simulink model "model_linear"  (R2021b)
settings: Solver=VariableStepAuto  StartTime=0.0  StopTime=10  RelTol=1e-3
undefined symbols (not defined in the file): D, J, ke, Kp, L, P, Q, R, Tp, U
libraries: slpidlib x1
settings Model: Creator=mateusz  LastModifiedBy=mateusz

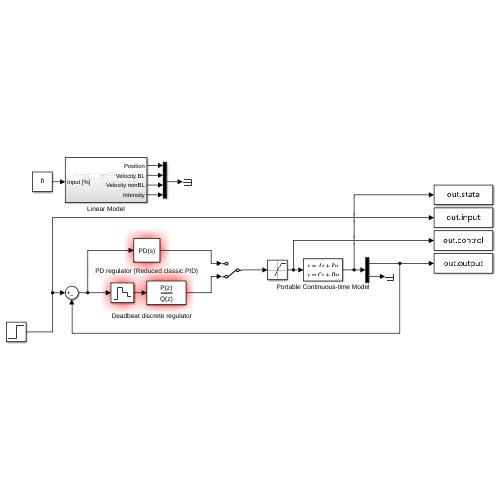
[thumbnail: Simulink's stored preview of the top-level diagram]
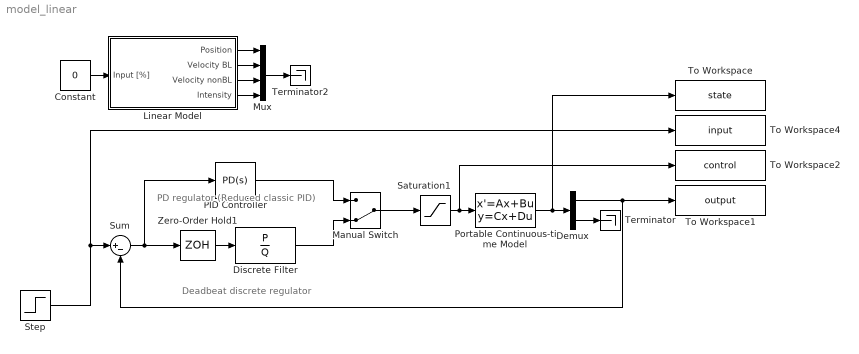
== system model_linear ==
  note: Deadbeat discrete regulator
  note: PD regulator (Reduced classic PID)
  Constant : Constant  Value=0
  Demux : Demux  Outputs=2
  Discrete Filter : DiscreteFilter  Numerator=P  Denominator=Q
  Linear Model : Subsystem
  Manual Switch : ManualSwitch  CurrentSetting=0
  Mux : Mux
  PID Controller : slpidlib/PID Controller  Controller=PD  Form=Parallel  TimeDomain=Continuous-time  UseExternalTs=off  SampleTime=-1  IntegratorMethod=Forward Euler  FilterMethod=Forward Euler  ControllerParametersSource=internal  P=Kp  I=0.000002  D=.667*Kp  UseFilter=on  N=100  TunerSelectOption=Transfer Function Based (PID Tuner App)  InitialConditionSource=internal  InitialConditionForIntegrator=0  InitialConditionForFilter=0  DifferentiatorICPrevScaledInput=0  ExternalReset=none  TrackingMode=off  Kt=1  LimitOutput=off  SatLimitsSource=internal  UpperSaturationLimit=inf  LowerSaturationLimit=-inf  LinearizeAsGain=on  AntiWindupMode=none  Kb=1  POutMin=[]  POutMax=[]  IOutMin=[]  IOutMax=[]  DOutMin=[]  DOutMax=[]  NOutMin=[]  NOutMax=[]  SumOutMin=[]  SumOutMax=[]  SaturationOutMin=[]  SaturationOutMax=[]  PParamMin=[]  PParamMax=[]  IParamMin=[]  IParamMax=[]  DParamMin=[]  DParamMax=[]  NParamMin=[]  NParamMax=[]  KbParamMin=[]  KbParamMax=[]  KtParamMin=[]  KtParamMax=[]  KbOutMin=[]  KbOutMax=[]  KtOutMin=[]  KtOutMax=[]  IntegratorOutMin=[]  IntegratorOutMax=[]  FilterOutMin=[]  FilterOutMax=[]  SumI1OutMin=[]  SumI1OutMax=[]  SumI2OutMin=[]  SumI2OutMax=[]  SumI3OutMin=[]  SumI3OutMax=[]  SumI4OutMin=[]  SumI4OutMax=[]  SumDOutMin=[]  SumDOutMax=[]  DifferentiatorOutMin=[]  DifferentiatorOutMax=[]  FilterDiffOutCoefMin=[]  FilterDiffOutCoefMax=[]  ReciprocalOutMin=[]  ReciprocalOutMax=[]  SumDenOutMin=[]  SumDenOutMax=[]  SumNumOutMin=[]  SumNumOutMax=[]  DivideOutMin=[]  DivideOutMax=[]  UdiffTsProdOutMin=[]  UdiffTsProdOutMax=[]  NTsProdOutMin=[]  NTsProdOutMax=[]  UintegralTsProdOutMin=[]  UintegralTsProdOutMax=[]  UngainTsProdOutMin=[]  UngainTsProdOutMax=[]  IntegratorContinuousStateAttributes=''  IntegratorStateMustResolveToSignalObject=off  IntegratorRTWStateStorageClass=Auto  FilterContinuousStateAttributes=''  FilterStateMustResolveToSignalObject=off  FilterRTWStateStorageClass=Auto  ParallelPVariant=InternalParameters  IdealPVariant=Disabled  IVariant=Disabled  DVariant=InternalParameters  IntegratorVariant=Disabled  SatVariant=Disabled  AWVariant=Disabled  PCopyVariant=Disabled  TRVariant=Disabled  FdbkBlocksVariant=Forward  IdealPFdbkVariant=Disabled  SatFdbkVariant=Disabled  DerivativeFilterVariant=ContFilter  NVariant=InternalParameters  NCopyVariant=Disabled  FilterICVariant=InternalICsFilter  IntegratorICVariant=Disabled  ExternalResetVariant=Disabled  TRSumVariant=Passthrough  SumFdbkVariant=Disabled  SumVariant=Sum_PD  TsampFilterVariant=InternalTs  TsampNgainVariant=Passthrough  TsampIntegralVariant=Disabled_SignalSpec  ExternalSaturationOutDataTypeStr=Inherit: Same as second input
  Portable Continuous-time Model : StateSpace  A=|  B=[0;0;0;2.59e4];  C=eye(4,4)  D=zeros(4,1)  InitialCondition=0
      | [0  1  0    0;
      |      0 -5  4.5  0;
      |      0  0 -0.7108*2  2*23.6012;
      |      0  0 -5.3898 -4040];
  Saturation1 : Saturate
  Step : Step  Time=0.5  After=6.28*25  SampleTime=0
  Sum : Sum  Inputs=|+-
  Terminator : Terminator
  Terminator2 : Terminator
  To Workspace : ToWorkspace  VariableName=state  SampleTime=-1
  To Workspace1 : ToWorkspace  VariableName=output  SampleTime=-1
  To Workspace2 : ToWorkspace  VariableName=control  SaveFormat=Structure With Time  SampleTime=0.001
  To Workspace4 : ToWorkspace  VariableName=input  SaveFormat=Structure With Time  SampleTime=-1
  Zero-Order Hold1 : ZeroOrderHold  SampleTime=Tp
  wires:
  Constant/1 -> Linear Model/1(Input [%])
  Linear Model/1(Position) -> Mux/1
  Linear Model/2(Velocity BL) -> Mux/2
  Linear Model/3(Velocity nonBL) -> Mux/3
  Linear Model/4(Intensity) -> Mux/4
  Portable Continuous-time Model/1 -> To Workspace/1, Demux/1
  Demux/1 -> To Workspace1/1, Sum/2
  Demux/2 -> Terminator/1
  Mux/1 -> Terminator2/1
  PID Controller/1 -> Manual Switch/1
  Zero-Order Hold1/1 -> Discrete Filter/1
  Manual Switch/1 -> Saturation1/1
  Discrete Filter/1 -> Manual Switch/2
  Saturation1/1 -> To Workspace2/1, Portable Continuous-time Model/1
  Step/1 -> To Workspace4/1, Sum/1
  Sum/1 -> PID Controller/1, Zero-Order Hold1/1

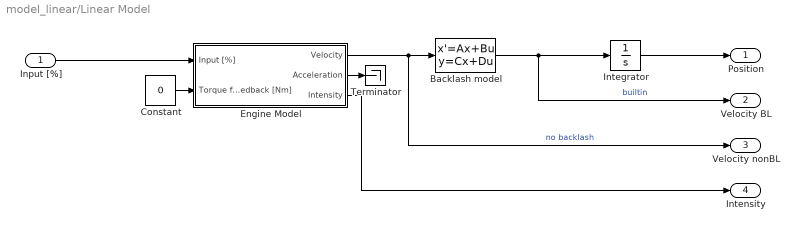
== system model_linear/Linear Model ==
  Input [%] : Inport
  Backlash model : StateSpace  A=[-5]  B=[4.5]  D=0  InitialCondition=0
  Constant : Constant  Value=0
  Engine Model : Subsystem
  Integrator : Integrator
  Terminator : Terminator
  Position : Outport
  Velocity BL : Outport  Port=2
  Velocity nonBL : Outport  Port=3
  Intensity : Outport  Port=4
  wires:
  Engine Model/3(Intensity) -> Intensity/1
  Input [%]/1 -> Engine Model/1(Input [%])
  Constant/1 -> Engine Model/2(Torque feedback [Nm])
  Engine Model/1(Velocity) -> Velocity nonBL/1, Backlash model/1  "no backlash"
  Integrator/1 -> Position/1
  Backlash model/1 -> Velocity BL/1, Integrator/1  "builtin"
  Engine Model/2(Acceleration) -> Terminator/1

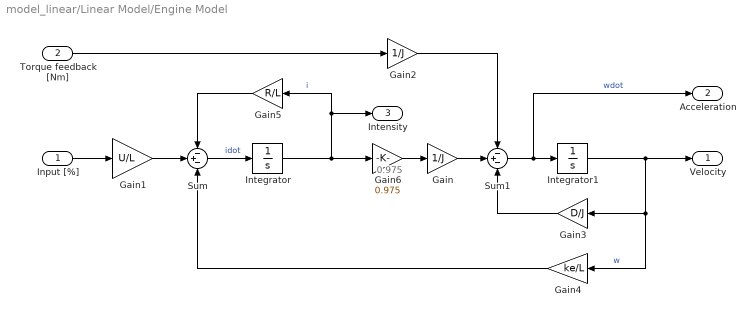
== system model_linear/Linear Model/Engine Model ==
  note: 0.975
  Input [%] : Inport
  Torque feedback [Nm] : Inport  Port=2
  Gain : Gain  Gain=1/J
  Gain1 : Gain  Gain=U/L
  Gain2 : Gain  Gain=1/J
  Gain3 : Gain  Gain=D/J
  Gain4 : Gain  Gain=ke/L
  Gain5 : Gain  Gain=R/L
  Gain6 : Gain  Gain=0.975
  Integrator : Integrator
  Integrator1 : Integrator
  Sum : Sum  Inputs=-+-
  Sum1 : Sum  Inputs=-+-
  Velocity : Outport
  Acceleration : Outport  Port=2
  Intensity : Outport  Port=3
  wires:
  Gain3/1 -> Sum1/3
  Input [%]/1 -> Gain1/1
  Gain4/1 -> Sum/3
  Gain6/1 -> Gain/1
  Gain/1 -> Sum1/2
  Gain5/1 -> Sum/1
  Sum/1 -> Integrator/1  "idot"
  Gain1/1 -> Sum/2
  Sum1/1 -> Acceleration/1, Integrator1/1  "wdot"
  Integrator/1 -> Gain6/1, Gain5/1, Intensity/1  "i"
  Integrator1/1 -> Velocity/1, Gain4/1, Gain3/1  "w"
  Torque feedback [Nm]/1 -> Gain2/1
  Gain2/1 -> Sum1/1
